simulink model "flightControlSystem"  (R2024b)
settings: Solver=ode3  StartTime=0  StopTime=TFinal  FixedStep=Ts  RelTol=1e-3  EnableMultiTasking=on
undefined symbols (not defined in the file): codertarget, Controller, DiscIntNeverNeededParam, Discrete, Estimator, g, gray, init, Sensors, Smin, T, Time, Ts, var_acc_angle_N, var_bias_gyr_N, var_gyro_p_N, Vehicle
libraries: simulink x39, slpidlib x4, ctrlSharedLib x4, sharedtransform x3, parrotlib x1
(part 3 of 3)

== matlab function flightControlSystem/Image Processing System/MATLAB Function ==
  data: redMask input; cleanMask output; kernelSize input
function cleanMask = BuildCenterBandMask(redMask, kernelSize)
%#codegen

H = 120;
W = 160;

temp = false(H,W);
cleanMask = false(H,W);

k = int32(kernelSize);
if k < 1
    k = int32(1);
end
if k > 31
    k = int32(31);
end

r = idivide(k, int32(2), 'floor');

% Horizontal erosion
for y = 1:H
    for x = 1:W
        keep = true;

        for dx = -r:r
            xx = x + dx;

            if xx < 1 || xx > W
                keep = false;
            else
                if redMask(y,xx) < 0.5
                    keep = false;
                end
            end
        end

        temp(y,x) = keep;
    end
end

% Vertical erosion
for y = 1:H
    for x = 1:W
        keep = true;

        for dy = -r:r
            yy = y + dy;

            if yy < 1 || yy > H
                keep = false;
            else
                if ~temp(yy,x)
                    keep = false;
                end
            end
        end

        cleanMask(y,x) = keep;
    end
end

end

== matlab function flightControlSystem/Control System/Controller/Position Controller/Position error transformation (Earth to Body frame) ==
  data: yaw input; xy_err_earth input; xy_err_body output
function xy_err_body = fcn(yaw,xy_err_earth)

transformation = [cos(yaw), sin(yaw); -sin(yaw),  cos(yaw)];
xy_err_body = transformation * xy_err_earth;


end

== matlab function flightControlSystem/Image Processing System/MATLAB Function1 ==
  data: cleanMask input; debugRGB output; v1_x input; v1_y input; v2_x input; v2_y input; v3_x input; v3_y input; valid1 input; valid2 input; valid3 input; dirX input; dirY input; useDir input
function debugRGB = DebugDrawVTP(cleanMask, v1_x, v1_y, v2_x, v2_y, v3_x, v3_y, valid1, valid2, valid3, dirX, dirY, useDir)
%#codegen

H = 120;
W = 160;

p0x = 80;
p0y = 60;

R1 = 18;
R2 = 32;
R3 = 48;
band = 3;

theta = 2.4;
cosHalf = cos(theta/2.0);

debugRGB = zeros(H,W,3,'uint8');

% draw ring/FoV search areas first
debugRGB = drawRing(debugRGB, R1, band, p0x, p0y, useDir, dirX, dirY, cosHalf, uint8([60 60 0]));
debugRGB = drawRing(debugRGB, R2, band, p0x, p0y, useDir, dirX, dirY, cosHalf, uint8([70 35 0]));
debugRGB = drawRing(debugRGB, R3, band, p0x, p0y, useDir, dirX, dirY, cosHalf, uint8([60 0 60]));

% draw cleanMask gray
for y = 1:H
    for x = 1:W
        if cleanMask(y,x) > 0.5
            debugRGB(y,x,1) = max(debugRGB(y,x,1), uint8(80));
            debugRGB(y,x,2) = max(debugRGB(y,x,2), uint8(80));
            debugRGB(y,x,3) = max(debugRGB(y,x,3), uint8(80));
        end
    end
end

% draw heading ray
if useDir > 0.5
    debugRGB = drawRay(debugRGB, p0x, p0y, dirX, dirY, int32(R3+8), uint8([0 120 255]));
end

% draw P0 red
debugRGB = drawSquare(debugRGB, int32(round(p0x)), int32(round(p0y)), uint8([255 0 0]));

% draw VTPs
if valid1 > 0.5
    debugRGB = drawSquare(debugRGB, int32(round(v1_x)), int32(round(v1_y)), uint8([255 255 0]));
end

if valid2 > 0.5
    debugRGB = drawSquare(debugRGB, int32(round(v2_x)), int32(round(v2_y)), uint8([255 128 0]));
end

if valid3 > 0.5
    debugRGB = drawSquare(debugRGB, int32(round(v3_x)), int32(round(v3_y)), uint8([255 0 255]));
end

end

function img = drawRing(img, R, band, p0x, p0y, useDir, dirX, dirY, cosHalf, color)
%#codegen

H = 120;
W = 160;

Rmin2 = double((R-band)*(R-band));
Rmax2 = double((R+band)*(R+band));

for y = 1:H
    for x = 1:W
        dx = double(x) - p0x;
        dy = double(y) - p0y;
        d2 = dx*dx + dy*dy;

        if d2 >= Rmin2 && d2 <= Rmax2
            accept = true;

            if useDir > 0.5
                d = sqrt(d2);
                if d > 0.001
                    ux = dx / d;
                    uy = dy / d;
                    dotv = ux*dirX + uy*dirY;

                    if dotv < cosHalf
                        accept = false;
                    end
                end
            end

            if accept
                img(y,x,1) = max(img(y,x,1), color(1));
                img(y,x,2) = max(img(y,x,2), color(2));
                img(y,x,3) = max(img(y,x,3), color(3));
            end
        end
    end
end

end

function img = drawRay(img, p0x, p0y, dirX, dirY, len, color)
%#codegen

H = 120;
W = 160;

for k = 0:len
    x = int32(round(p0x + dirX * double(k)));
    y = int32(round(p0y + dirY * double(k)));

    if x >= 1 && x <= W && y >= 1 && y <= H
        img(y,x,1) = color(1);
        img(y,x,2) = color(2);
        img(y,x,3) = color(3);
    end
end

end

function img = drawSquare(img, x, y, color)
%#codegen

H = 120;
W = 160;

for yy = y-2:y+2
    for xx = x-2:x+2
        if xx >= 1 && xx <= W && yy >= 1 && yy <= H
            img(yy,xx,1) = color(1);
            img(yy,xx,2) = color(2);
            img(yy,xx,3) = color(3);
        end
    end
end

end

== matlab function flightControlSystem/Image Processing System/MATLAB Function2 ==
  data: cleanMask input; v1_x output; prevDirX input; prevDirY input; v1_y output; v2_x output; v2_y output; v3_x output; v3_y output; valid1 output; valid2 output; valid3 output; dirX output; dirY output; useDir output
function [v1_x,v1_y,v2_x,v2_y,v3_x,v3_y,valid1,valid2,valid3,dirX,dirY,useDir] = MultiRingVTP(cleanMask, prevDirX, prevDirY)
%#codegen

p0x = 80;
p0y = 60;

R1 = 18;
R2 = 32;
R3 = 48;
band = 3;

theta = 2.4;
cosHalf = cos(theta/2.0);

pn = sqrt(prevDirX*prevDirX + prevDirY*prevDirY);

useDir = 0;
dirX = 0;
dirY = 0;

if pn > 0.5
    useDir = 1;
    dirX = prevDirX / pn;
    dirY = prevDirY / pn;
end

[v1_x,v1_y,valid1] = findVTP(cleanMask, R1, band, p0x, p0y, useDir, dirX, dirY, cosHalf);
[v2_x,v2_y,valid2] = findVTP(cleanMask, R2, band, p0x, p0y, useDir, dirX, dirY, cosHalf);
[v3_x,v3_y,valid3] = findVTP(cleanMask, R3, band, p0x, p0y, useDir, dirX, dirY, cosHalf);

end

function [vx,vy,valid] = findVTP(mask, R, band, p0x, p0y, useDir, dirX, dirY, cosHalf)
%#codegen

H = 120;
W = 160;

sumX = 0;
sumY = 0;
count = 0;

Rmin2 = double((R-band)*(R-band));
Rmax2 = double((R+band)*(R+band));

for y = 1:H
    for x = 1:W
        if mask(y,x) > 0.5
            dx = double(x) - p0x;
            dy = double(y) - p0y;
            d2 = dx*dx + dy*dy;

            if d2 >= Rmin2 && d2 <= Rmax2
                accept = true;

                if useDir > 0.5
                    d = sqrt(d2);
                    if d > 0.001
                        ux = dx / d;
                        uy = dy / d;
                        dotv = ux*dirX + uy*dirY;

                        if dotv < cosHalf
                            accept = false;
                        end
                    end
                end

                if accept
                    sumX = sumX + double(x);
                    sumY = sumY + double(y);
                    count = count + 1;
                end
            end
        end
    end
end

if count > 0
    vx = sumX / double(count);
    vy = sumY / double(count);
    valid = 1;
else
    vx = p0x;
    vy = p0y;
    valid = 0;
end

end

== matlab function flightControlSystem/Control System/Path Planning/MATLAB Function ==
  data: v1_x input; target_x output; v1_y input; v2_x input; v2_y input; v3_x input; v3_y input; valid1 input; valid2 input; valid3 input; target_y output; targetValid output; targetLevel output; cornerMode input
function [target_x, target_y, targetValid, targetLevel] = SelectVTP(v1_x, v1_y, v2_x, v2_y, v3_x, v3_y, valid1, valid2, valid3, cornerMode)
%#codegen

target_x = 80;
target_y = 60;
targetValid = 0;
targetLevel = 0;

if cornerMode > 0.5
    % Corner mode:
    % Use close target first to avoid cutting inside the corner.
    if valid1 > 0.5
        target_x = v1_x;
        target_y = v1_y;
        targetValid = 1;
        targetLevel = 1;

    elseif valid2 > 0.5
        target_x = v2_x;
        target_y = v2_y;
        targetValid = 1;
        targetLevel = 2;

    elseif valid3 > 0.5
        target_x = v3_x;
        target_y = v3_y;
        targetValid = 1;
        targetLevel = 3;
    end

else
    % Normal mode:
    % V2 is the default lookahead target.
    if valid2 > 0.5
        target_x = v2_x;
        target_y = v2_y;
        targetValid = 1;
        targetLevel = 2;

    elseif valid1 > 0.5
        target_x = v1_x;
        target_y = v1_y;
        targetValid = 1;
        targetLevel = 1;

    elseif valid3 > 0.5
        target_x = v3_x;
        target_y = v3_y;
        targetValid = 1;
        targetLevel = 3;
    end
end

end

== matlab function flightControlSystem/Control System/Path Planning/MATLAB Function1 ==
  data: target_x input; dirX output; target_y input; targetValid input; prevDirX input; prevDirY input; dirY output; dirValid output
function [dirX, dirY, dirValid] = UpdatePrevDir(target_x, target_y, targetValid, prevDirX, prevDirY)
%#codegen

p0x = 80;
p0y = 60;

dirX = 0;
dirY = 0;
dirValid = 0;

if targetValid < 0.5
    return;
end

% Direction from camera center to selected VTP target
dx = target_x - p0x;
dy = target_y - p0y;

n = sqrt(dx*dx + dy*dy);

if n < 3
    return;
end

newX = dx / n;
newY = dy / n;

pn = sqrt(prevDirX*prevDirX + prevDirY*prevDirY);

% If previous direction is unknown, use new direction directly
if pn < 0.5
    dirX = newX;
    dirY = newY;
    dirValid = 1;
    return;
end

prevX = prevDirX / pn;
prevY = prevDirY / pn;

dotv = prevX*newX + prevY*newY;

% Turn-gated smoothing
if dotv > 0.85
    alpha = 0.8;   % almost straight
elseif dotv > 0.3
    alpha = 0.5;   % moderate turn
elseif dotv > -0.2
    alpha = 0.25;  % sharp turn
else
    alpha = 0.1;   % possible bad target or reverse direction
end

mixX = alpha*newX + (1-alpha)*prevX;
mixY = alpha*newY + (1-alpha)*prevY;

mn = sqrt(mixX*mixX + mixY*mixY);

if mn > 0.001
    dirX = mixX / mn;
    dirY = mixY / mn;
    dirValid = 1;
end

end
